simulink model "myfir_filter_unfolded"  (R2020b)
settings: Solver=VariableStepAuto  StartTime=0.0  StopTime=10.0  RelTol=1e-3
settings Model: Creator=Francesco  LastModifiedBy=gianp
settings DataIOCC: ReturnWorkspaceOutputs=off
settings DebuggingCC: ArithmeticOperatorsInVariantConditions=warning
settings SFSimCC: CustomCodeUndefinedFunction=UseInterfaceOnly

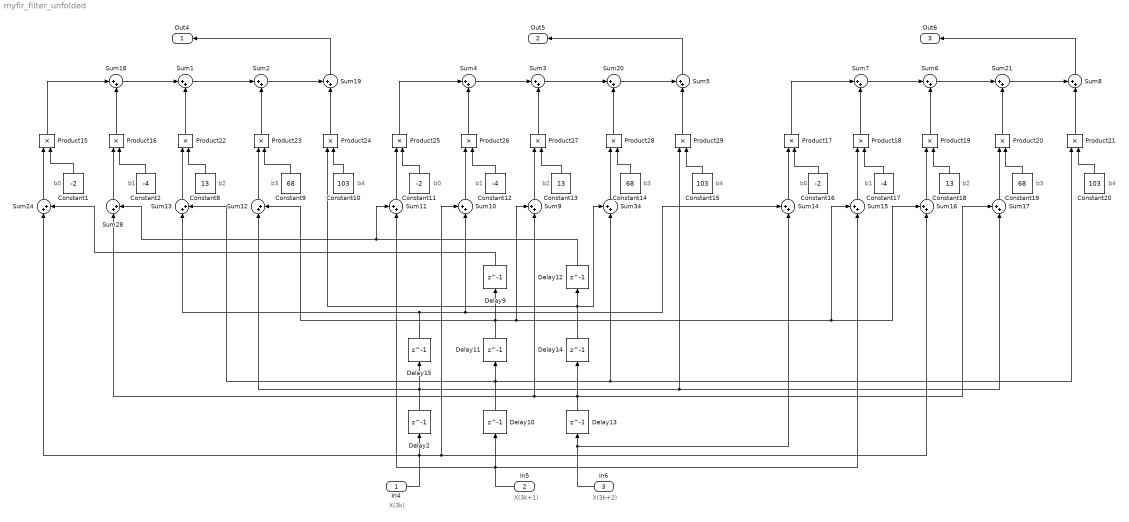
== system myfir_filter_unfolded ==
  note: X(3k+2)
  note: X(3k+1)
  note: X(3k)
  note: b0
  note: b1
  note: b2
  note: b3
  note: b4
  note: b2
  note: b3
  note: b0
  note: b1
  note: b0
  note: b2
  note: b3
  note: b4
  note: b1
  note: b4
  In4 : Inport
  In5 : Inport  Port=2
  In6 : Inport  Port=3
  Constant1 : Constant  Tag=b0  Description=b0  Value=-2
  Constant10 : Constant  Tag=b0  Description=b0  Value=103
  Constant11 : Constant  Tag=b0  Description=b0  Value=-2
  Constant12 : Constant  Tag=b0  Description=b0  Value=-4
  Constant13 : Constant  Tag=b0  Description=b0  Value=13
  Constant14 : Constant  Tag=b0  Description=b0  Value=68
  Constant15 : Constant  Tag=b0  Description=b0  Value=103
  Constant16 : Constant  Tag=b0  Description=b0  Value=-2
  Constant17 : Constant  Tag=b0  Description=b0  Value=-4
  Constant18 : Constant  Tag=b0  Description=b0  Value=13
  Constant19 : Constant  Tag=b0  Description=b0  Value=68
  Constant2 : Constant  Tag=b0  Description=b0  Value=-4
  Constant20 : Constant  Tag=b0  Description=b0  Value=103
  Constant8 : Constant  Tag=b0  Description=b0  Value=13
  Constant9 : Constant  Tag=b0  Description=b0  Value=68
  Delay{2,9..15} (8 alike) : Delay  DelayLength=1  InitialCondition=0
  Product{15..29} (15 alike) : Product
  Sum{1..4,6..7,12..13,18,20..21,24,28} (13 alike) : Sum  Inputs=|++
  Sum{5,8..11,14..17,19,34} (11 alike) : Sum  Inputs=++|
  Out4 : Outport  SignalName=y(3k)  VectorParamsAs1DForOutWhenUnconnected=off
  Out5 : Outport  Port=2  SignalName=y(3k+1)  VectorParamsAs1DForOutWhenUnconnected=off
  Out6 : Outport  Port=3  SignalName=y(3k+2)  VectorParamsAs1DForOutWhenUnconnected=off
  wires:
  In5/1 -> Sum11/2, Sum15/2, Delay10/1
  In4/1 -> Sum16/2, Sum10/1, Delay2/1, Sum24/1
  In6/1 -> Sum14/2, Delay13/1
  Delay10/1 -> Product21/1, Sum34/2, Sum13/2, Delay11/1
  Delay13/1 -> Delay14/1, Sum17/1, Sum28/1, Sum9/2
  Delay11/1 -> Sum15/1, Sum16/1, Sum9/1, Delay9/1, Sum12/2
  Constant1/1 -> Product15/2
  Delay9/1 -> Sum24/2
  Sum24/1 -> Product15/1
  Constant2/1 -> Product16/2
  Delay14/1 -> Delay12/1, Sum34/1, Product24/1
  Delay12/1 -> Sum11/1, Sum28/2
  Sum28/1 -> Product16/1
  Product16/1 -> Sum18/2
  Constant8/1 -> Product22/2
  Delay2/1 -> Sum17/2, Product29/1, Sum12/1, Delay15/1
  Sum13/1 -> Product22/1
  Delay15/1 -> Sum10/2, Sum14/1, Sum13/1
  Constant9/1 -> Product23/2
  Sum12/1 -> Product23/1
  Constant10/1 -> Product24/2
  Constant11/1 -> Product25/2
  Sum11/1 -> Product25/1
  Sum10/1 -> Product26/1
  Constant13/1 -> Product27/2
  Sum9/1 -> Product27/1
  Constant14/1 -> Product28/2
  Constant12/1 -> Product26/2
  Sum34/1 -> Product28/1
  Constant15/1 -> Product29/2
  Constant19/1 -> Product20/2
  Constant18/1 -> Product19/2
  Sum17/1 -> Product20/1
  Sum16/1 -> Product19/1
  Constant17/1 -> Product18/2
  Constant16/1 -> Product17/2
  Constant20/1 -> Product21/2
  Sum14/1 -> Product17/1
  Sum15/1 -> Product18/1
  Product15/1 -> Sum18/1
  Sum18/1 -> Sum1/1
  Product22/1 -> Sum1/2
  Sum1/1 -> Sum2/1
  Product23/1 -> Sum2/2
  Sum2/1 -> Sum19/1
  Product24/1 -> Sum19/2
  Sum19/1 -> Out4/1
  Product29/1 -> Sum5/2
  Sum4/1 -> Sum3/1
  Product28/1 -> Sum20/2
  Product27/1 -> Sum3/2
  Product25/1 -> Sum4/1
  Sum20/1 -> Sum5/1
  Product26/1 -> Sum4/2
  Sum3/1 -> Sum20/1
  Sum5/1 -> Out5/1
  Product21/1 -> Sum8/2
  Sum7/1 -> Sum6/1
  Product19/1 -> Sum6/2
  Product17/1 -> Sum7/1
  Sum21/1 -> Sum8/1
  Product18/1 -> Sum7/2
  Sum6/1 -> Sum21/1
  Sum8/1 -> Out6/1
  Product20/1 -> Sum21/2
